simulink model "main"  (R2024b)
settings: Solver=ode45  StartTime=0.0  StopTime=40  MaxStep=0.001  RelTol=1e-3
InitFcn:
  | initial
values from neighbouring files (symbols this model uses):
  a_max = 3.5    [constraint.m]    (also in initial.m)
  a_min = -3.5    [constraint.m]    (also in initial.m)
  airDensityKgpm3 = 1.225    [initial.m]
  areaM2 = 2.5    [initial.m]
  coeffDrag = 0.28    [initial.m]
  dt_pid = 1e-2    (= 0.01)    [initial.m]
  gravityMps2 = 9.81    [initial.m]
  massKg = 2500    [initial.m]
  massKg1 = 2400    [initial.m]
  mu = 0.7    [constraint.m]    (also in initial.m; objective.m; sfunction_sid.m)
  pole_placement = -0.9    [initial.m]
  v0 = 10    [initial.m]    (also in sfunction_sid.m = block.InputPort(1).Data)
undefined symbols (not defined in the file or in its folder): DiscIntNeverNeededParam
libraries: simulink x1, eeStairGenerator x1
settings Model: PauseTimes=0.2  Creator=siddhik  LastModifiedBy=siddhik
settings SolverCC: ZeroCrossAlgorithm=Adaptive
settings DebuggingCC: IgnoredZcDiagnostic=none

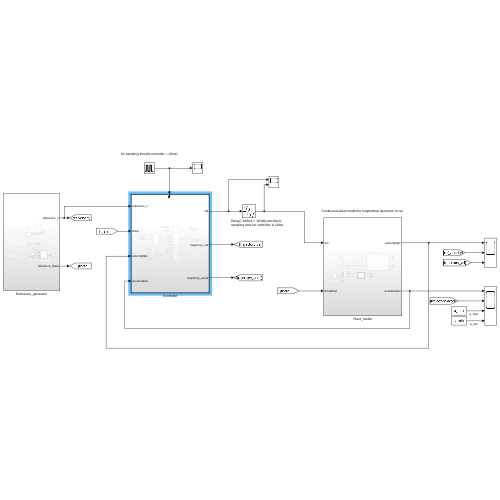
[thumbnail: Simulink's stored preview of the top-level diagram]
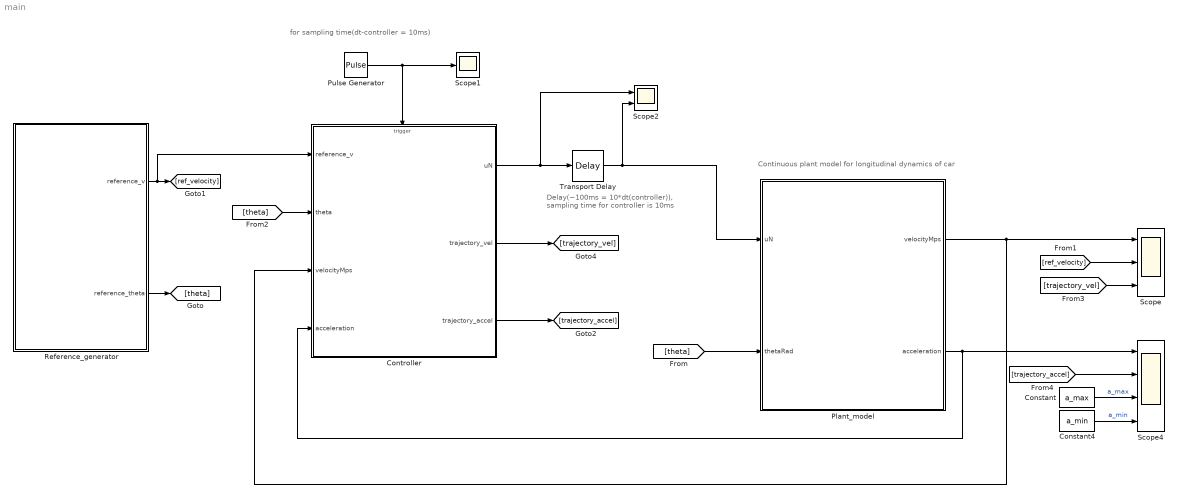
== system main ==
  note: Continuous plant model for longitudinal dynamics of car
  note: for sampling time(dt-controller = 10ms)
  note: Delay(~100ms = 10*dt(controller)),
      | sampling time for controller is 10ms
  Constant : Constant  Value=a_max
  Constant4 : Constant  Value=a_min
  Controller : Subsystem
  Plant_model : Subsystem
  Pulse Generator : DiscretePulseGenerator  PulseType=Time based  Period=0.01  PulseWidth=10
  Reference_generator : Subsystem
  Scope : Scope  NumInputPorts=3
  Scope1 : Scope
  Scope2 : Scope  NumInputPorts=2
  Scope4 : Scope  NumInputPorts=4
  Transport Delay : TransportDelay  DelayTime=0.1
  wires:
  Pulse Generator/1 -> Scope1/1, Controller/Trigger
  Plant_model/1(velocityMps) -> Controller/3(velocityMps), Scope/1
  Reference_generator/1(reference_v) -> [ref_velocity], Controller/1(reference_v)
  Reference_generator/2(reference_theta) -> [theta]
  [theta] -> Plant_model/2(thetaRad)
  [ref_velocity] -> Scope/2
  [theta] -> Controller/2(theta)
  Plant_model/2(acceleration) -> Controller/4(acceleration), Scope4/1
  Controller/1(uN) -> Transport Delay/1, Scope2/1
  Transport Delay/1 -> Plant_model/1(uN), Scope2/2
  Controller/2(trajectory_vel) -> [trajectory_vel]
  Controller/3(trajectory_accel) -> [trajectory_accel]
  [trajectory_accel] -> Scope4/2
  [trajectory_vel] -> Scope/3
  Constant/1 -> Scope4/3  "a_max"
  Constant4/1 -> Scope4/4  "a_min"

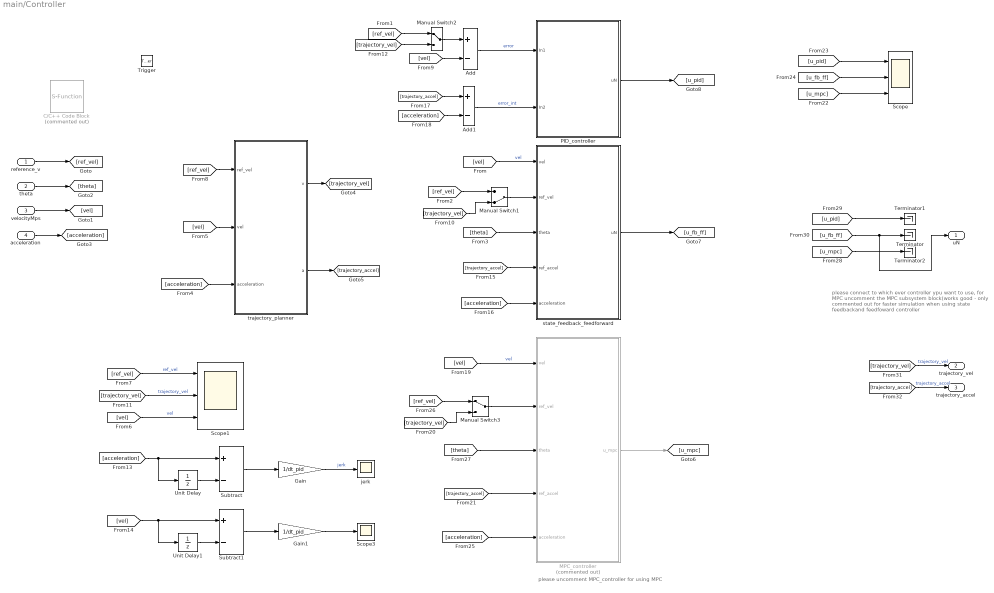
== system main/Controller ==
  note: please uncomment MPC_controller for using MPC
  note: please connect to which ever controller ypu want to use,
      | for MPC uncomment the MPC subsystem block(works good
      | - only commented out for faster simulation when using
      | state feedbackand feedfoward controller
  reference_v : Inport
  theta : Inport  Port=2
  velocityMps : Inport  Port=3
  acceleration : Inport  Port=4
  Trigger : TriggerPort  VariantControl=(inherit)  PortDimensions=1
  Add : Sum  Inputs=+-
  Add1 : Sum  Inputs=+-
  C/C++ Code Block : S-Function  Commented=on  SFunctionDeploymentMode=off  EnableBusSupport=off  mask(S-Function Builder){}
      mask help: Simulink:masks:SFunctionBuilder_MD
      mask init:
      | val = [[.9  0.75 0.75 1 1 .9 .9 1]',[1 1 0.75 0.75 .9 .9 1 .9]'];try , sys = get_param(gcb,'SfunBuilderFcnName');if isempty(sys), sys = get_param(gcb,'FunctionName'); end,catch, sys = get_param(gcb,'FunctionName'); end
      settings: CopyFcn=set_param(gcbh,'LinkStatus','none')  OpenFcn=sfunctionwizard(gcbh)
      mask Display:
      | plot(val(:,1),val(:,2))
      | disp(sys)
  Gain : Gain  Gain=1/dt_pid
  Gain1 : Gain  Gain=1/dt_pid
  MPC_controller : Subsystem  Commented=on
  Manual Switch1 : ManualSwitch  CurrentSetting=0
  Manual Switch2 : ManualSwitch
  Manual Switch3 : ManualSwitch
  PID_controller : Subsystem
  Scope : Scope  NumInputPorts=3
  Scope1 : Scope  NumInputPorts=3
  Scope3 : Scope
  Subtract : Sum  Inputs=+-
  Subtract1 : Sum  Inputs=+-
  Terminator : Terminator
  Terminator1 : Terminator
  Terminator2 : Terminator
  Unit Delay : UnitDelay  SampleTime=-1  HasFrameUpgradeWarning=on
  Unit Delay1 : UnitDelay  SampleTime=-1  HasFrameUpgradeWarning=on
  jerk : Scope
  state_feedback_feedforward : Subsystem
  trajectory_planner : Subsystem
  uN : Outport
  trajectory_vel : Outport  Port=2
  trajectory_accel : Outport  Port=3
  wires:
  reference_v/1 -> [ref_vel]
  velocityMps/1 -> [vel]
  Add/1 -> PID_controller/1(In1)  "error"
  [vel] -> state_feedback_feedforward/1(vel)  "vel"
  theta/1 -> [theta]
  PID_controller/1(uN) -> [u_pid]
  [theta] -> state_feedback_feedforward/3(theta)
  [vel] -> Scope1/3  "vel"
  [ref_vel] -> Scope1/1  "ref_vel"
  acceleration/1 -> [acceleration]
  [vel] -> Add/2
  [ref_vel] -> trajectory_planner/1(ref_vel)
  [acceleration] -> trajectory_planner/3(acceleration)
  [vel] -> trajectory_planner/2(vel)
  trajectory_planner/1(v) -> [trajectory_vel]
  [ref_vel] -> Manual Switch1/1
  [trajectory_vel] -> Manual Switch1/2
  Manual Switch1/1 -> state_feedback_feedforward/2(ref_vel)
  [trajectory_vel] -> Scope1/2  "trajectory_vel"
  Manual Switch2/1 -> Add/1
  [trajectory_vel] -> Manual Switch2/2
  [ref_vel] -> Manual Switch2/1
  [acceleration] -> Unit Delay/1, Subtract/1
  Unit Delay/1 -> Subtract/2
  Subtract/1 -> Gain/1
  Gain/1 -> jerk/1  "jerk"
  [vel] -> Unit Delay1/1, Subtract1/1
  Unit Delay1/1 -> Subtract1/2
  Gain1/1 -> Scope3/1
  Subtract1/1 -> Gain1/1
  trajectory_planner/2(a) -> [trajectory_accel]
  [trajectory_accel] -> state_feedback_feedforward/4(ref_accel)
  [acceleration] -> state_feedback_feedforward/5(acceleration)
  [trajectory_accel] -> Add1/1
  [acceleration] -> Add1/2
  Add1/1 -> PID_controller/2(In2)  "error_int"
  [u_mpc] -> Scope/3
  state_feedback_feedforward/1(uN) -> [u_fb_ff]
  [u_fb_ff] -> Scope/2
  [u_pid] -> Scope/1
  Manual Switch3/1 -> MPC_controller/2(ref_vel)
  [vel] -> MPC_controller/1(vel)  "vel"
  [ref_vel] -> Manual Switch3/1
  [trajectory_vel] -> Manual Switch3/2
  [trajectory_accel] -> MPC_controller/4(ref_accel)
  [theta] -> MPC_controller/3(theta)
  [acceleration] -> MPC_controller/5(acceleration)
  MPC_controller/1(u_mpc) -> [u_mpc]
  [u_pid] -> Terminator1/1
  [u_mpc] -> Terminator2/1
  [trajectory_vel] -> trajectory_vel/1  "trajectory_vel"
  [trajectory_accel] -> trajectory_accel/1  "trajectory_accel"
  [u_fb_ff] -> uN/1, Terminator/1

== system main/Plant_model ==
  note: not used, just used for open-loop
  note: This is just for initialization
  uN : Inport
  thetaRad : Inport  Port=2
  Clock : Clock
  "Initialization " : Subsystem
  Initialization 1 : Subsystem
  Model : ModelReference  ModelNameDialog=car_longitudinal_dynamics_plant.slx  SimulationMode=Normal  ModelReferenceVersion=5.4
  Scope : Scope
  Scope1 : Scope
  Scope2 : Scope  NumInputPorts=2
  Switch : Switch  Criteria=u2 > Threshold  Threshold=0.2  SaturateOnIntegerOverflow=off  InputSameDT=off
  plant_model : Subsystem
  velocityMps : Outport
  acceleration : Outport  Port=2
  wires:
  thetaRad/1 -> plant_model/2(thetaRad), Model/2
  Model/1 -> velocityMps/1  "velocity"
  Model/2 -> acceleration/1  "acceleration"
  plant_model/1(velocityMps) -> Scope/1
  plant_model/2(acceleration) -> Scope1/1
  uN/1 -> Scope2/1, Switch/1
  Clock/1 -> Switch/2
  Switch/1 -> Model/1
  "Initialization "/1(Out1) -> Scope2/2, Switch/3
  Initialization 1/1(uN) -> plant_model/1(uN)

== system main/Reference_generator ==
  note: not used, just for verification
  note: for negative slope
  note: for positive slope
  Clock : Clock
  Constant2 : Constant  Value=2
  MATLAB Function : MATLAB Function  Commented=on  TreatAsAtomicUnit=on
  MATLAB Function1 : MATLAB Function  TreatAsAtomicUnit=on
  Repeating Sequence : simulink/Sources/Repeating Sequence  rep_seq_t=[0 0.2 0.2001 8 8.001 16 16.001 30 30.001 50 50.001 55 55.001 70]  rep_seq_y=[0 0 10 10 20 20 50 50 30 30 50 50 30 30]
  Scope : Scope
  Scope1 : Scope
  Stair Generator : eeStairGenerator/Stair Generator  Commented=on  LabelModeActiveChoice=Discrete  TimeInput=[0.0 1 3 10 20]  AmplitudeInput=[0 10 20 50 50]  SampleTime=1e-2  RepeatPattern=off  OutDataTypeStr=double
      settings: LibrarySourceBlock=ee_sl_lib/General Control/Stair Generator
  theta_slope : Step  Before=20*pi/180  After=20*pi/180  SampleTime=0
  theta_slope1 : Step  Commented=on  Before=-20*pi/180  After=-20*pi/180  SampleTime=0
  velocity_ref : Step  Time=10  Before=v0  After=20  SampleTime=0
  velocity_ref1 : Step  Time=10  Before=20  After=50  SampleTime=0
  velocity_ref2 : Step  Commented=on  Time=10  After=10  SampleTime=0
  reference_v : Outport
  reference_theta : Outport  Port=2
  wires:
  theta_slope/1 -> reference_theta/1
  velocity_ref/1 -> MATLAB Function1/1(v0)
  velocity_ref1/1 -> MATLAB Function1/2(vf)
  Clock/1 -> MATLAB Function1/4(dt)
  Constant2/1 -> MATLAB Function1/3(a_max)
  MATLAB Function1/1(v) -> Scope/1
  Repeating Sequence/1 -> reference_v/1, Scope1/1

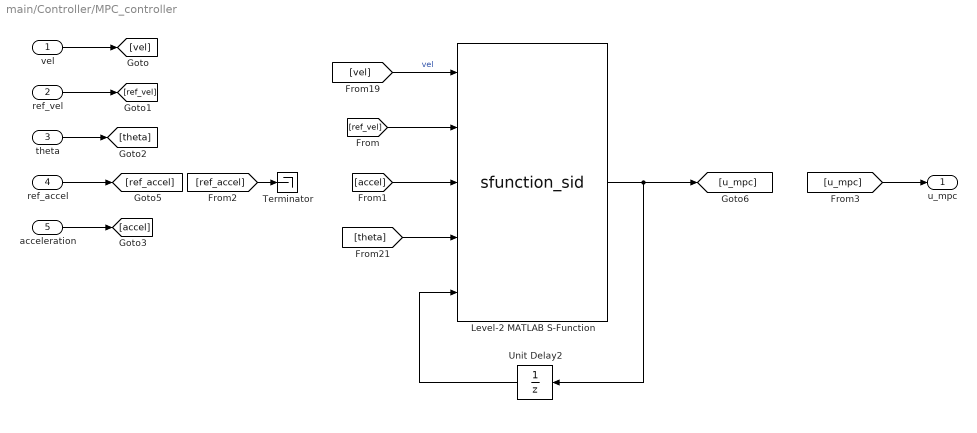
== system main/Controller/MPC_controller ==
  vel : Inport
  ref_vel : Inport  Port=2
  theta : Inport  Port=3
  ref_accel : Inport  Port=4
  acceleration : Inport  Port=5
  Level-2 MATLAB S-Function : M-S-Function  FunctionName=sfunction_sid
  Terminator : Terminator
  Unit Delay2 : UnitDelay  InitialCondition=8838  SampleTime=-1  HasFrameUpgradeWarning=on
  u_mpc : Outport
  wires:
  [ref_vel] -> Level-2 MATLAB S-Function/2
  [accel] -> Level-2 MATLAB S-Function/3
  Level-2 MATLAB S-Function/1 -> [u_mpc], Unit Delay2/1
  [vel] -> Level-2 MATLAB S-Function/1  "vel"
  [theta] -> Level-2 MATLAB S-Function/4
  Unit Delay2/1 -> Level-2 MATLAB S-Function/5
  vel/1 -> [vel]
  ref_vel/1 -> [ref_vel]
  acceleration/1 -> [accel]
  ref_accel/1 -> [ref_accel]
  theta/1 -> [theta]
  [ref_accel] -> Terminator/1
  [u_mpc] -> u_mpc/1

== system main/Controller/PID_controller ==
  In1 : Inport
  In2 : Inport  Port=2
  Discrete-Time Integrator : DiscreteIntegrator  SampleTime=-1  ICPrevOutput=DiscIntNeverNeededParam  ICPrevScaledInput=DiscIntNeverNeededParam
  Gain : Gain  Gain=10000
  Gain1 : Gain  Gain=0
  Gain2 : Gain  Gain=500
  Gain3 : Gain  Gain=1000
  Scope : Scope  NumInputPorts=2
  Sum : Sum  Inputs=++++
  d_term : UnitDelay  SampleTime=-1  HasFrameUpgradeWarning=on
  integrator : Subsystem
  uN : Outport
  wires:
  Gain/1 -> Sum/2
  d_term/1 -> Sum/1
  Sum/1 -> uN/1
  In1/1 -> Gain2/1, Gain1/1, Gain/1
  Gain1/1 -> d_term/1
  Gain2/1 -> integrator/1(Ki*error), Discrete-Time Integrator/1
  Discrete-Time Integrator/1 -> Scope/2
  integrator/1(ki_sum) -> Sum/3, Scope/1
  In2/1 -> Gain3/1
  Gain3/1 -> Sum/4

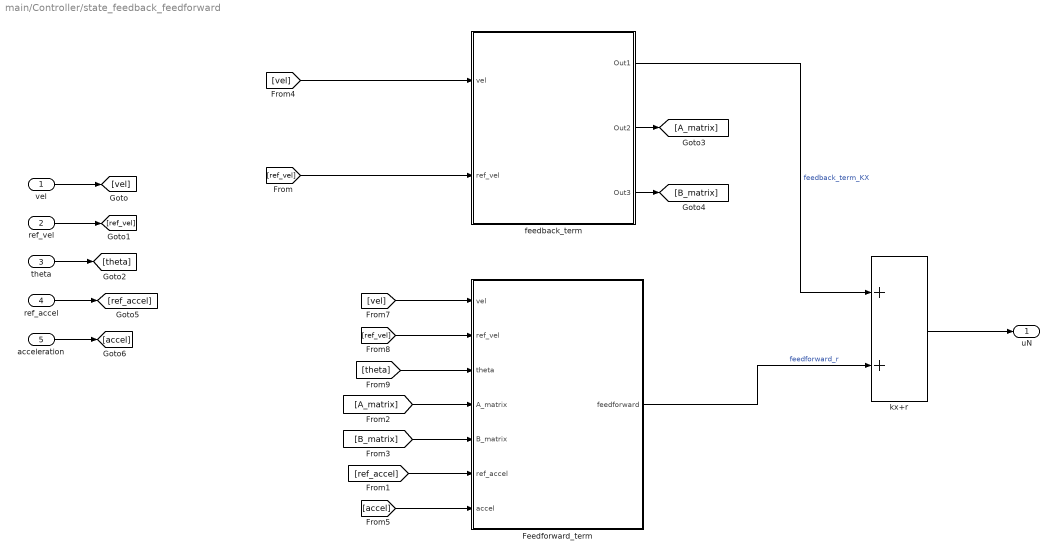
== system main/Controller/state_feedback_feedforward ==
  vel : Inport
  ref_vel : Inport  Port=2
  theta : Inport  Port=3
  ref_accel : Inport  Port=4
  acceleration : Inport  Port=5
  Feedforward_term : Subsystem
  feedback_term : Subsystem
  kx+r : Sum
  uN : Outport
  wires:
  vel/1 -> [vel]
  ref_vel/1 -> [ref_vel]
  theta/1 -> [theta]
  kx+r/1 -> uN/1
  Feedforward_term/1(feedforward) -> kx+r/2  "feedforward_r"
  [vel] -> Feedforward_term/1(vel)
  [ref_vel] -> Feedforward_term/2(ref_vel)
  [theta] -> Feedforward_term/3(theta)
  [A_matrix] -> Feedforward_term/4(A_matrix)
  [B_matrix] -> Feedforward_term/5(B_matrix)
  [vel] -> feedback_term/1(vel)
  feedback_term/1(Out1) -> kx+r/1  "feedback_term_KX"
  [ref_vel] -> feedback_term/2(ref_vel)
  feedback_term/2(Out2) -> [A_matrix]
  feedback_term/3(Out3) -> [B_matrix]
  ref_accel/1 -> [ref_accel]
  [ref_accel] -> Feedforward_term/6(ref_accel)
  acceleration/1 -> [accel]
  [accel] -> Feedforward_term/7(accel)

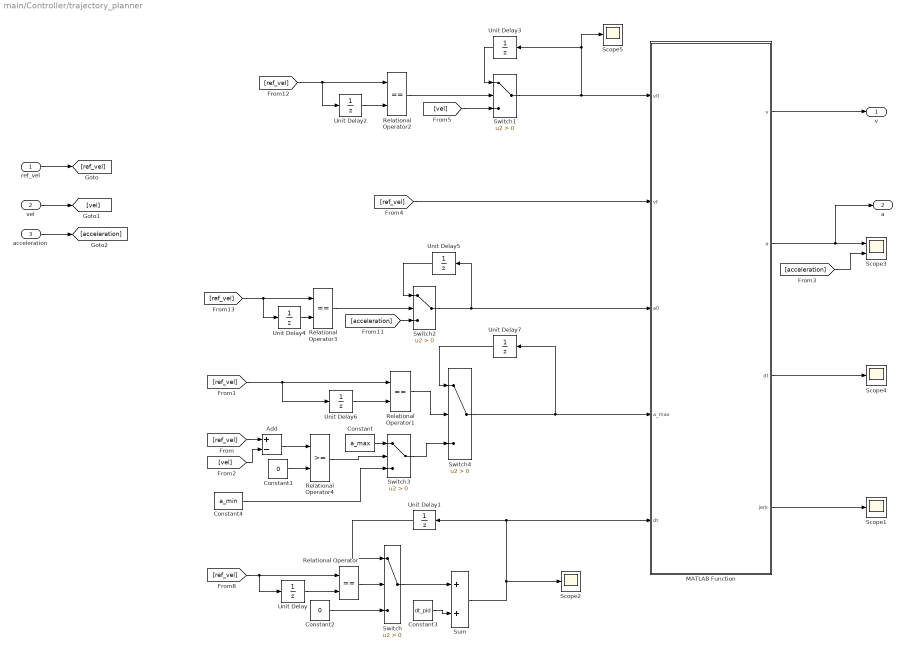
== system main/Controller/trajectory_planner ==
  ref_vel : Inport
  vel : Inport  Port=2
  acceleration : Inport  Port=3
  Add : Sum  Inputs=+-
  Constant : Constant  Value=a_max
  Constant1 : Constant  Value=0
  Constant2 : Constant  Value=0
  Constant3 : Constant  Value=dt_pid
  Constant4 : Constant  Value=a_min
  MATLAB Function : MATLAB Function  TreatAsAtomicUnit=on
  Relational Operator{,1..3} (4 alike) : RelationalOperator  Operator===  OutDataTypeStr=boolean  RndMeth=Simplest  InputSameDT=off
  Relational Operator4 : RelationalOperator  OutDataTypeStr=boolean  RndMeth=Simplest  InputSameDT=off
  Scope{1..2,4..5} (4 alike) : Scope
  Scope3 : Scope  NumInputPorts=2
  Sum : Sum
  Switch{,1..4} (5 alike) : Switch  Criteria=u2 > Threshold  SaturateOnIntegerOverflow=off  InputSameDT=off
  Unit Delay{,2,4,6} (4 alike) : UnitDelay  SampleTime=-1  HasFrameUpgradeWarning=on
  Unit Delay{1,3,5,7} (4 alike) : UnitDelay  InitialCondition=v0  SampleTime=-1  HasFrameUpgradeWarning=on
  v : Outport
  a : Outport  Port=2
  wires:
  Switch2/1 -> Unit Delay5/1, MATLAB Function/3(a0)
  Sum/1 -> Unit Delay1/1, MATLAB Function/5("dt "), Scope2/1
  [vel] -> Switch1/3
  [ref_vel] -> Unit Delay2/1, Relational Operator2/1
  MATLAB Function/2(a) -> a/1, Scope3/1
  Unit Delay/1 -> Relational Operator/2
  [acceleration] -> Switch2/3
  MATLAB Function/1(v) -> v/1
  MATLAB Function/3(dt) -> Scope4/1
  Relational Operator2/1 -> Switch1/2
  Switch/1 -> Sum/1
  Unit Delay4/1 -> Relational Operator3/2
  Constant2/1 -> Switch/3
  Relational Operator3/1 -> Switch2/2
  Constant3/1 -> Sum/2
  Unit Delay3/1 -> Switch1/1
  Switch1/1 -> Scope5/1, Unit Delay3/1, MATLAB Function/1(v0)
  [ref_vel] -> Unit Delay/1, Relational Operator/1
  Unit Delay2/1 -> Relational Operator2/2
  [ref_vel] -> MATLAB Function/2(vf)
  [ref_vel] -> Unit Delay4/1, Relational Operator3/1
  Unit Delay1/1 -> Switch/1
  Unit Delay5/1 -> Switch2/1
  ref_vel/1 -> [ref_vel]
  vel/1 -> [vel]
  acceleration/1 -> [acceleration]
  Relational Operator/1 -> Switch/2
  [ref_vel] -> Unit Delay6/1, Relational Operator1/1
  Unit Delay6/1 -> Relational Operator1/2
  Relational Operator1/1 -> Switch4/2
  Switch4/1 -> Unit Delay7/1, MATLAB Function/4(a_max)
  Unit Delay7/1 -> Switch4/1
  [ref_vel] -> Add/1
  [vel] -> Add/2
  Add/1 -> Relational Operator4/1
  Constant1/1 -> Relational Operator4/2
  Switch3/1 -> Switch4/3
  Relational Operator4/1 -> Switch3/2
  Constant/1 -> Switch3/1
  Constant4/1 -> Switch3/3
  [acceleration] -> Scope3/2
  MATLAB Function/4(jerk) -> Scope1/1

== system main/Plant_model/Initialization  ==
  Constant1 : Constant  Value=0
  Manual Switch1 : ManualSwitch
  theta_slope1 : Step  Before=20*pi/180  After=20*pi/180  SampleTime=0
  u_0_equilibium1 : Subsystem
  u_0_equilibium2 : Subsystem
  Out1 : Outport
  wires:
  u_0_equilibium1/1(u_0) -> Manual Switch1/1
  Constant1/1 -> u_0_equilibium2/1(vel), u_0_equilibium1/1(vel)
  u_0_equilibium2/1(u_0) -> Manual Switch1/2
  theta_slope1/1 -> u_0_equilibium2/2(theta), u_0_equilibium1/2(theta)
  Manual Switch1/1 -> Out1/1

== system main/Plant_model/Initialization 1 ==
  Constant1 : Constant  Value=0
  Manual Switch1 : ManualSwitch
  theta_slope1 : Step  Before=20*pi/180  After=20*pi/180  SampleTime=0
  u_0_equilibium1 : Subsystem
  u_0_equilibium2 : Subsystem
  uN : Outport
  wires:
  u_0_equilibium1/1(u_0) -> Manual Switch1/1
  Constant1/1 -> u_0_equilibium2/1(vel), u_0_equilibium1/1(vel)
  u_0_equilibium2/1(u_0) -> Manual Switch1/2
  theta_slope1/1 -> u_0_equilibium2/2(theta), u_0_equilibium1/2(theta)
  Manual Switch1/1 -> uN/1

== system main/Plant_model/plant_model ==
  uN : Inport
  thetaRad : Inport  Port=2
  car_longitudinal_dynamics : Subsystem
  velocityMps : Outport
  acceleration : Outport  Port=2
  wires:
  uN/1 -> car_longitudinal_dynamics/1(uN)
  thetaRad/1 -> car_longitudinal_dynamics/2(thetaRad)
  car_longitudinal_dynamics/1(velocityMps) -> velocityMps/1
  car_longitudinal_dynamics/2(acceleration) -> acceleration/1

== system main/Controller/PID_controller/integrator ==
  Ki*error : Inport
  Gain : Gain  Gain=dt_pid
  Sum : Sum
  Unit Delay : UnitDelay  SampleTime=-1  HasFrameUpgradeWarning=on
  Unit Delay1 : UnitDelay  SampleTime=-1  HasFrameUpgradeWarning=on
  ki_sum : Outport
  wires:
  Unit Delay/1 -> Sum/1
  Sum/1 -> Unit Delay/1, Unit Delay1/1
  Ki*error/1 -> Gain/1
  Gain/1 -> Sum/2
  Unit Delay1/1 -> ki_sum/1

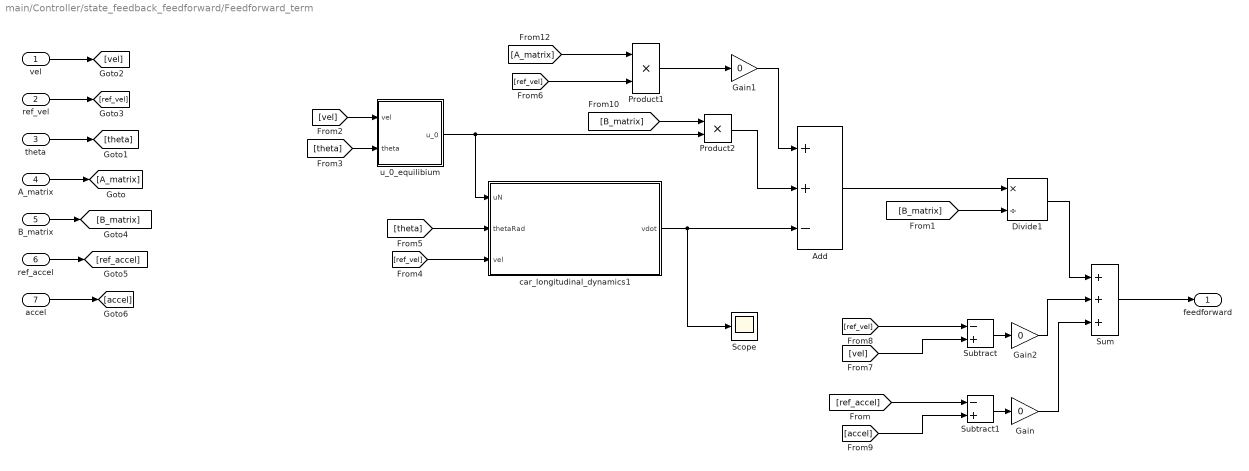
== system main/Controller/state_feedback_feedforward/Feedforward_term ==
  vel : Inport
  ref_vel : Inport  Port=2
  theta : Inport  Port=3
  A_matrix : Inport  Port=4
  B_matrix : Inport  Port=5
  ref_accel : Inport  Port=6
  accel : Inport  Port=7
  Add : Sum  Inputs=++-
  Divide1 : Product  Inputs=*/
  Gain : Gain  Gain=0
  Gain1 : Gain  Gain=0
  Gain2 : Gain  Gain=0
  Product1 : Product
  Product2 : Product
  Scope : Scope
  Subtract : Sum  Inputs=-+
  Subtract1 : Sum  Inputs=-+
  Sum : Sum  Inputs=+++
  car_longitudinal_dynamics1 : Subsystem
  u_0_equilibium : Subsystem
  feedforward : Outport
  wires:
  car_longitudinal_dynamics1/1(vdot) -> Scope/1, Add/3
  [B_matrix] -> Divide1/2
  Product2/1 -> Add/2
  [A_matrix] -> Product1/1
  [theta] -> u_0_equilibium/2(theta)
  [ref_vel] -> Product1/2
  u_0_equilibium/1(u_0) -> Product2/2, car_longitudinal_dynamics1/1(uN)
  Product1/1 -> Gain1/1
  [theta] -> car_longitudinal_dynamics1/2(thetaRad)
  [ref_vel] -> car_longitudinal_dynamics1/3(vel)
  [B_matrix] -> Product2/1
  Add/1 -> Divide1/1
  [vel] -> u_0_equilibium/1(vel)
  Gain1/1 -> Add/1
  A_matrix/1 -> [A_matrix]
  theta/1 -> [theta]
  vel/1 -> [vel]
  ref_vel/1 -> [ref_vel]
  B_matrix/1 -> [B_matrix]
  ref_accel/1 -> [ref_accel]
  accel/1 -> [accel]
  [ref_vel] -> Subtract/1
  Sum/1 -> feedforward/1
  Divide1/1 -> Sum/1
  [vel] -> Subtract/2
  [ref_accel] -> Subtract1/1
  [accel] -> Subtract1/2
  Subtract1/1 -> Gain/1
  Subtract/1 -> Gain2/1
  Gain/1 -> Sum/3
  Gain2/1 -> Sum/2

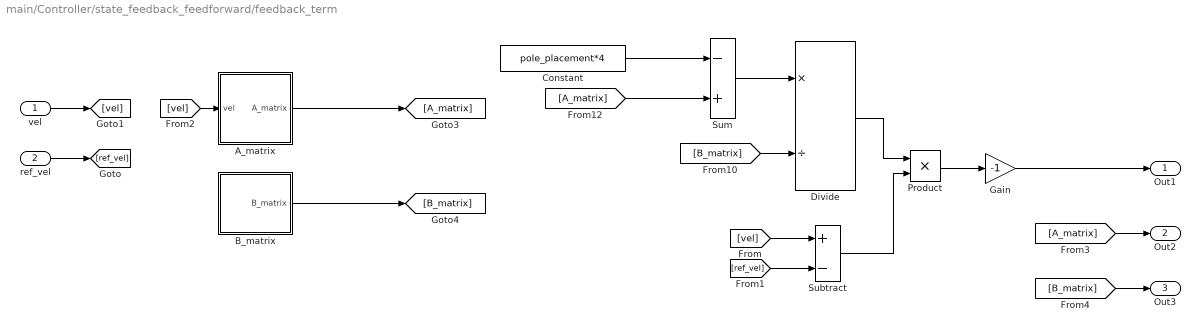
== system main/Controller/state_feedback_feedforward/feedback_term ==
  vel : Inport
  ref_vel : Inport  Port=2
  A_matrix : Subsystem
  B_matrix : Subsystem
  Constant : Constant  Value=pole_placement*4
  Divide : Product  Inputs=*/
  Gain : Gain  Gain=-1
  Product : Product
  Subtract : Sum  Inputs=+-
  Sum : Sum  Inputs=-+
  Out1 : Outport
  Out2 : Outport  Port=2
  Out3 : Outport  Port=3
  wires:
  B_matrix/1(B_matrix) -> [B_matrix]
  [ref_vel] -> Subtract/2
  [B_matrix] -> Divide/2
  Sum/1 -> Divide/1
  Gain/1 -> Out1/1
  Product/1 -> Gain/1
  [A_matrix] -> Sum/2
  Constant/1 -> Sum/1
  A_matrix/1(A_matrix) -> [A_matrix]
  [vel] -> Subtract/1
  Subtract/1 -> Product/2
  Divide/1 -> Product/1
  ref_vel/1 -> [ref_vel]
  vel/1 -> [vel]
  [vel] -> A_matrix/1(vel)
  [A_matrix] -> Out2/1
  [B_matrix] -> Out3/1

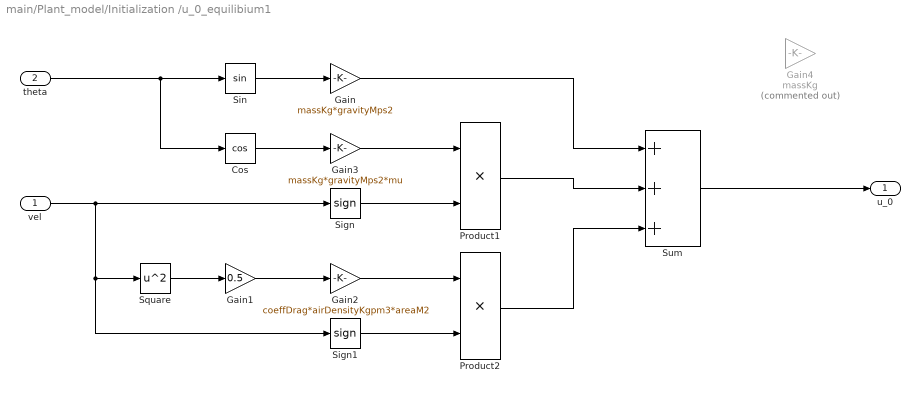
== system main/Plant_model/Initialization /u_0_equilibium1 ==
  vel : Inport
  theta : Inport  Port=2
  Cos : Trigonometry  Operator=cos
  Gain : Gain  Gain=massKg*gravityMps2
      settings: AttributesFormatString=%<Gain>
  Gain1 : Gain  Gain=0.5
      settings: AttributesFormatString=%<Gain>
  Gain2 : Gain  Gain=coeffDrag*airDensityKgpm3*areaM2
      settings: AttributesFormatString=%<Gain>
  Gain3 : Gain  Gain=massKg*gravityMps2*mu
      settings: AttributesFormatString=%<Gain>
  Gain4 : Gain  Commented=on  Gain=massKg
      settings: AttributesFormatString=%<Gain>
  Product1 : Product
  Product2 : Product
  Sign : Signum
  Sign1 : Signum
  Sin : Trigonometry
  Square : Math  Operator=square
  Sum : Sum  Inputs=+++
  u_0 : Outport
  wires:
  Gain1/1 -> Gain2/1
  Cos/1 -> Gain3/1
  Sin/1 -> Gain/1
  theta/1 -> Sin/1, Cos/1
  Sign1/1 -> Product2/2
  Gain3/1 -> Product1/1
  Gain2/1 -> Product2/1
  Sign/1 -> Product1/2
  Square/1 -> Gain1/1
  vel/1 -> Square/1, Sign1/1, Sign/1
  Gain/1 -> Sum/1
  Product1/1 -> Sum/2
  Product2/1 -> Sum/3
  Sum/1 -> u_0/1

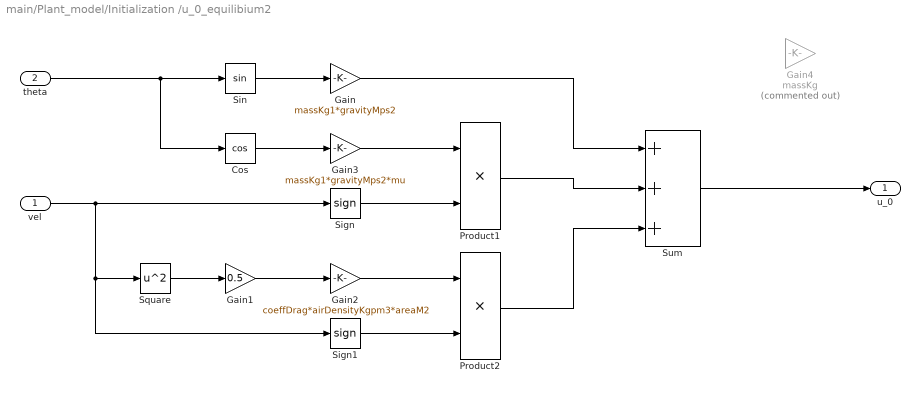
== system main/Plant_model/Initialization /u_0_equilibium2 ==
  vel : Inport
  theta : Inport  Port=2
  Cos : Trigonometry  Operator=cos
  Gain : Gain  Gain=massKg1*gravityMps2
      settings: AttributesFormatString=%<Gain>
  Gain1 : Gain  Gain=0.5
      settings: AttributesFormatString=%<Gain>
  Gain2 : Gain  Gain=coeffDrag*airDensityKgpm3*areaM2
      settings: AttributesFormatString=%<Gain>
  Gain3 : Gain  Gain=massKg1*gravityMps2*mu
      settings: AttributesFormatString=%<Gain>
  Gain4 : Gain  Commented=on  Gain=massKg
      settings: AttributesFormatString=%<Gain>
  Product1 : Product
  Product2 : Product
  Sign : Signum
  Sign1 : Signum
  Sin : Trigonometry
  Square : Math  Operator=square
  Sum : Sum  Inputs=+++
  u_0 : Outport
  wires:
  Gain1/1 -> Gain2/1
  Cos/1 -> Gain3/1
  Sin/1 -> Gain/1
  theta/1 -> Sin/1, Cos/1
  Sign1/1 -> Product2/2
  Gain3/1 -> Product1/1
  Gain2/1 -> Product2/1
  Sign/1 -> Product1/2
  Square/1 -> Gain1/1
  vel/1 -> Square/1, Sign1/1, Sign/1
  Gain/1 -> Sum/1
  Product1/1 -> Sum/2
  Product2/1 -> Sum/3
  Sum/1 -> u_0/1

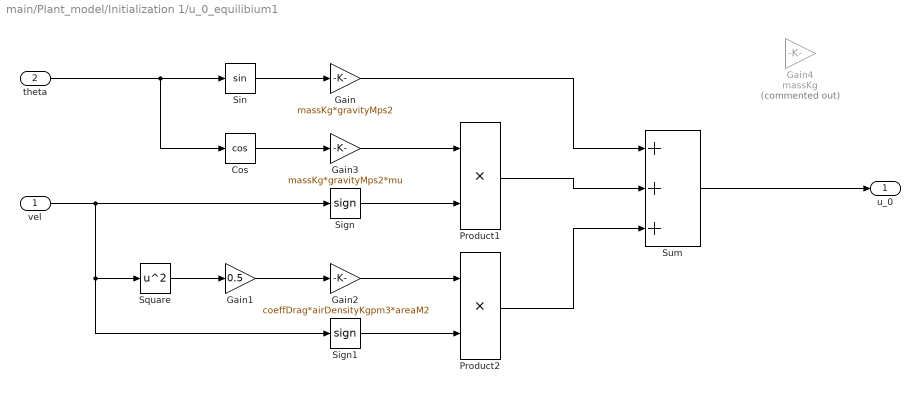
== system main/Plant_model/Initialization 1/u_0_equilibium1 ==
  vel : Inport
  theta : Inport  Port=2
  Cos : Trigonometry  Operator=cos
  Gain : Gain  Gain=massKg*gravityMps2
      settings: AttributesFormatString=%<Gain>
  Gain1 : Gain  Gain=0.5
      settings: AttributesFormatString=%<Gain>
  Gain2 : Gain  Gain=coeffDrag*airDensityKgpm3*areaM2
      settings: AttributesFormatString=%<Gain>
  Gain3 : Gain  Gain=massKg*gravityMps2*mu
      settings: AttributesFormatString=%<Gain>
  Gain4 : Gain  Commented=on  Gain=massKg
      settings: AttributesFormatString=%<Gain>
  Product1 : Product
  Product2 : Product
  Sign : Signum
  Sign1 : Signum
  Sin : Trigonometry
  Square : Math  Operator=square
  Sum : Sum  Inputs=+++
  u_0 : Outport
  wires:
  Gain1/1 -> Gain2/1
  Cos/1 -> Gain3/1
  Sin/1 -> Gain/1
  theta/1 -> Sin/1, Cos/1
  Sign1/1 -> Product2/2
  Gain3/1 -> Product1/1
  Gain2/1 -> Product2/1
  Sign/1 -> Product1/2
  Square/1 -> Gain1/1
  vel/1 -> Square/1, Sign1/1, Sign/1
  Gain/1 -> Sum/1
  Product1/1 -> Sum/2
  Product2/1 -> Sum/3
  Sum/1 -> u_0/1

== system main/Plant_model/Initialization 1/u_0_equilibium2 ==
  vel : Inport
  theta : Inport  Port=2
  Cos : Trigonometry  Operator=cos
  Gain : Gain  Gain=massKg1*gravityMps2
      settings: AttributesFormatString=%<Gain>
  Gain1 : Gain  Gain=0.5
      settings: AttributesFormatString=%<Gain>
  Gain2 : Gain  Gain=coeffDrag*airDensityKgpm3*areaM2
      settings: AttributesFormatString=%<Gain>
  Gain3 : Gain  Gain=massKg1*gravityMps2*mu
      settings: AttributesFormatString=%<Gain>
  Gain4 : Gain  Commented=on  Gain=massKg
      settings: AttributesFormatString=%<Gain>
  Product1 : Product
  Product2 : Product
  Sign : Signum
  Sign1 : Signum
  Sin : Trigonometry
  Square : Math  Operator=square
  Sum : Sum  Inputs=+++
  u_0 : Outport
  wires:
  Gain1/1 -> Gain2/1
  Cos/1 -> Gain3/1
  Sin/1 -> Gain/1
  theta/1 -> Sin/1, Cos/1
  Sign1/1 -> Product2/2
  Gain3/1 -> Product1/1
  Gain2/1 -> Product2/1
  Sign/1 -> Product1/2
  Square/1 -> Gain1/1
  vel/1 -> Square/1, Sign1/1, Sign/1
  Gain/1 -> Sum/1
  Product1/1 -> Sum/2
  Product2/1 -> Sum/3
  Sum/1 -> u_0/1

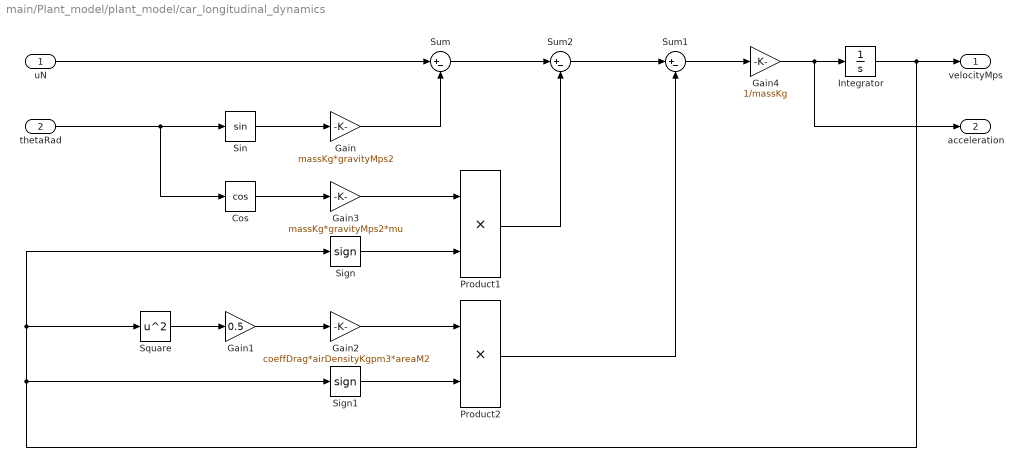
== system main/Plant_model/plant_model/car_longitudinal_dynamics ==
  uN : Inport
  thetaRad : Inport  Port=2
  Cos : Trigonometry  Operator=cos
  Gain : Gain  Gain=massKg*gravityMps2
      settings: AttributesFormatString=%<Gain>
  Gain1 : Gain  Gain=0.5
      settings: AttributesFormatString=%<Gain>
  Gain2 : Gain  Gain=coeffDrag*airDensityKgpm3*areaM2
      settings: AttributesFormatString=%<Gain>
  Gain3 : Gain  Gain=massKg*gravityMps2*mu
      settings: AttributesFormatString=%<Gain>
  Gain4 : Gain  Gain=1/massKg
      settings: AttributesFormatString=%<Gain>
  Integrator : Integrator
  Product1 : Product
  Product2 : Product
  Sign : Signum
  Sign1 : Signum
  Sin : Trigonometry
  Square : Math  Operator=square
  Sum : Sum  Inputs=|+-
  Sum1 : Sum  Inputs=|+-
  Sum2 : Sum  Inputs=|+-
  velocityMps : Outport
  acceleration : Outport  Port=2
  wires:
  uN/1 -> Sum/1
  thetaRad/1 -> Sin/1, Cos/1
  Gain1/1 -> Gain2/1
  Gain2/1 -> Product2/1
  Integrator/1 -> velocityMps/1, Sign1/1, Sign/1, Square/1
  Product2/1 -> Sum1/2
  Sum2/1 -> Sum1/1
  Sum/1 -> Sum2/1
  Sin/1 -> Gain/1
  Gain/1 -> Sum/2
  Cos/1 -> Gain3/1
  Gain3/1 -> Product1/1
  Product1/1 -> Sum2/2
  Sum1/1 -> Gain4/1
  Gain4/1 -> acceleration/1, Integrator/1
  Square/1 -> Gain1/1
  Sign/1 -> Product1/2
  Sign1/1 -> Product2/2

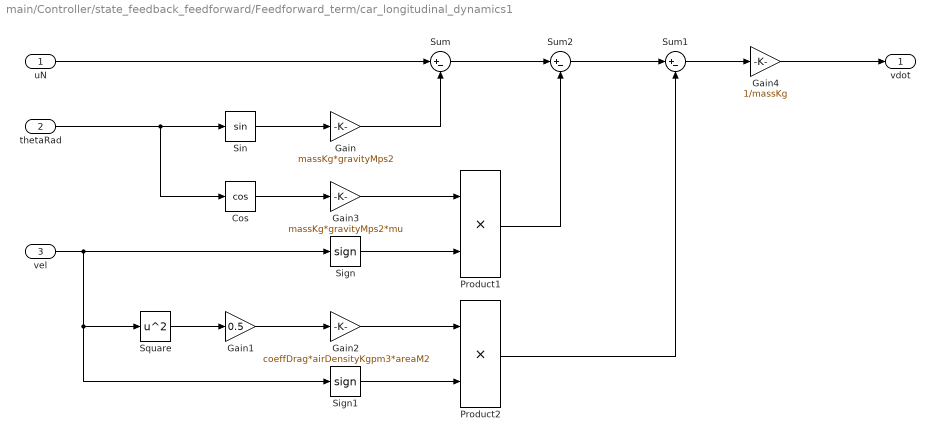
== system main/Controller/state_feedback_feedforward/Feedforward_term/car_longitudinal_dynamics1 ==
  uN : Inport
  thetaRad : Inport  Port=2
  vel : Inport  Port=3
  Cos : Trigonometry  Operator=cos
  Gain : Gain  Gain=massKg*gravityMps2
      settings: AttributesFormatString=%<Gain>
  Gain1 : Gain  Gain=0.5
      settings: AttributesFormatString=%<Gain>
  Gain2 : Gain  Gain=coeffDrag*airDensityKgpm3*areaM2
      settings: AttributesFormatString=%<Gain>
  Gain3 : Gain  Gain=massKg*gravityMps2*mu
      settings: AttributesFormatString=%<Gain>
  Gain4 : Gain  Gain=1/massKg
      settings: AttributesFormatString=%<Gain>
  Product1 : Product
  Product2 : Product
  Sign : Signum
  Sign1 : Signum
  Sin : Trigonometry
  Square : Math  Operator=square
  Sum : Sum  Inputs=|+-
  Sum1 : Sum  Inputs=|+-
  Sum2 : Sum  Inputs=|+-
  vdot : Outport
  wires:
  uN/1 -> Sum/1
  thetaRad/1 -> Sin/1, Cos/1
  Gain1/1 -> Gain2/1
  Gain2/1 -> Product2/1
  Gain4/1 -> vdot/1
  Product2/1 -> Sum1/2
  Sum2/1 -> Sum1/1
  Sum/1 -> Sum2/1
  Sin/1 -> Gain/1
  Gain/1 -> Sum/2
  Cos/1 -> Gain3/1
  Gain3/1 -> Product1/1
  Product1/1 -> Sum2/2
  Sum1/1 -> Gain4/1
  Square/1 -> Gain1/1
  Sign/1 -> Product1/2
  Sign1/1 -> Product2/2
  vel/1 -> Sign/1, Sign1/1, Square/1

== system main/Controller/state_feedback_feedforward/Feedforward_term/u_0_equilibium ==
  vel : Inport
  theta : Inport  Port=2
  Cos : Trigonometry  Operator=cos
  Gain : Gain  Gain=massKg*gravityMps2
      settings: AttributesFormatString=%<Gain>
  Gain1 : Gain  Gain=0.5
      settings: AttributesFormatString=%<Gain>
  Gain2 : Gain  Gain=coeffDrag*airDensityKgpm3*areaM2
      settings: AttributesFormatString=%<Gain>
  Gain3 : Gain  Gain=massKg*gravityMps2*mu
      settings: AttributesFormatString=%<Gain>
  Gain4 : Gain  Commented=on  Gain=massKg
      settings: AttributesFormatString=%<Gain>
  Product1 : Product
  Product2 : Product
  Sign : Signum
  Sign1 : Signum
  Sin : Trigonometry
  Square : Math  Operator=square
  Sum : Sum  Inputs=+++
  u_0 : Outport
  wires:
  Gain1/1 -> Gain2/1
  Cos/1 -> Gain3/1
  Sin/1 -> Gain/1
  theta/1 -> Sin/1, Cos/1
  Sign1/1 -> Product2/2
  Gain3/1 -> Product1/1
  Gain2/1 -> Product2/1
  Sign/1 -> Product1/2
  Square/1 -> Gain1/1
  vel/1 -> Square/1, Sign1/1, Sign/1
  Gain/1 -> Sum/1
  Product1/1 -> Sum/2
  Product2/1 -> Sum/3
  Sum/1 -> u_0/1

== system main/Controller/state_feedback_feedforward/feedback_term/A_matrix ==
  vel : Inport
  Gain : Gain  Gain=-1
  Gain4 : Gain  Gain=1/massKg
      settings: AttributesFormatString=%<Gain>
  Gain6 : Gain  Gain=coeffDrag*airDensityKgpm3*areaM2
      settings: AttributesFormatString=%<Gain>
  Product3 : Product
  Sign2 : Signum
  A_matrix : Outport
  wires:
  vel/1 -> Gain6/1, Sign2/1
  Sign2/1 -> Product3/2
  Gain6/1 -> Product3/1
  Product3/1 -> Gain4/1
  Gain4/1 -> Gain/1
  Gain/1 -> A_matrix/1

== system main/Controller/state_feedback_feedforward/feedback_term/B_matrix ==
  Constant : Constant  Value=1/massKg
  B_matrix : Outport
  wires:
  Constant/1 -> B_matrix/1

== matlab function main/Controller/trajectory_planner/MATLAB Function ==
  data: v0 input; v output; vf input; a0 input; a_max input; dt input; a output; dt output; jerk output
function [v, a, dt, jerk] = fcn(v0, vf, a0, a_max, dt)
%#codegen
% Computes velocity (v) and acceleration (a) at time dt
% v = A + B*t + C*t*t + D*t*t*t;
% a = B + 2*C*t + 3*D*t*t;
    if abs(v0 - vf) < 1e-3
        v = vf;
        a = 0;
        jerk = 0;
        return;
    end
    

    % Compute final time based on constraints
    tf = 6 * (vf - v0) / (a0 + 4 * a_max);

    % Polynomial coefficients
    A = v0;                           
    B = a0;                           
    C = (4 * a_max - 3 * a0) / (2 * tf);         
    D = (2 * a0 - 4 * a_max) / (3 * tf^2);        

    % Clamp dt to tf to avoid overshooting
    if dt > tf
        dt = tf;
    end

    % Compute velocity and acceleration at time dt
    v = A + B * dt + C * dt^2 + D * dt^3;
    a = B + 2 * C * dt + 3 * D * dt^2;
    jerk = 2 * C + 6 * D*dt;
end

== matlab function main/Reference_generator/MATLAB Function ==
  data: u input; y output
function y = fcn(u)
%#codegen

y = u;

== matlab function main/Reference_generator/MATLAB Function1 ==
  data: v0 input; v output; vf input; a_max input; dt input
function v = fcn(v0, vf, a_max, dt)
%#codegen
% v = a + b*t + c*t^2 + d*t^3;
% a = b + 2*c*t + 3*d*t^2;

%if abs(v0 - vf) < 0.1
    % If the difference between initial and final velocity is small
  % v = vf;
%else
    % Polynomial coefficients for the trajectory
    a = v0;
    b = 0;
    tf = 3 * (vf - v0) / (2 * a_max);  % Time to reach vf
    c = 2 * a_max / (tf);
    d = -4*a_max / (3*tf^2);
    if(tf<dt)
        dt = tf;
    end
    % Compute the position at time dt
    v = a + b * dt + c * dt^2 + d * dt^3;
%end
